simulink model "Brushless"  (R2020a)
settings: Solver=ode23  StartTime=0.0  StopTime=10.0  MaxStep=1e-2  RelTol=1e-3
undefined symbols (not defined in the file): CQ, I, Ke, Om, R, Ra, tau, V0, w_cm, zeta
libraries: fmu_me_lib x1, simulink x1
settings Model: Creator=Bob  LastModifiedBy=meagh
settings SFSimCC: CustomCodeUndefinedFunction=UseInterfaceOnly

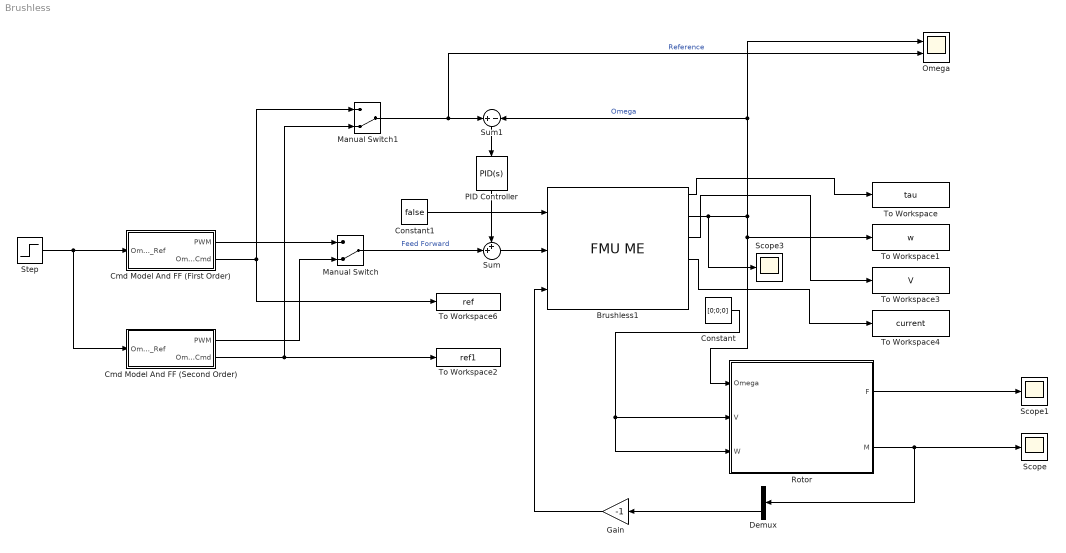
== system Brushless ==
  Brushless1 : fmu_me_lib/FMU ME  Description=Simulates an FMU for Model Exchange 1.0 or Model Exchange 2.0.  dummy=0
  Cmd Model And FF (First Order) : Subsystem
  Cmd Model And FF (Second Order) : Subsystem
  Constant : Constant  Value=[0;0;0]
  Constant1 : Constant  Value=false  OutDataTypeStr=boolean
  Demux : Demux  Outputs=3
  Gain : Gain  Gain=-1
  Manual Switch : ManualSwitch  CurrentSetting=0
  Manual Switch1 : ManualSwitch  CurrentSetting=0
  Omega : Scope  NumInputPorts=2
  PID Controller : simulink/Continuous/PID Controller  Controller=PID  Form=Parallel  TimeDomain=Continuous-time  UseExternalTs=off  SampleTime=-1  IntegratorMethod=Forward Euler  FilterMethod=Forward Euler  ControllerParametersSource=internal  P=0.0184*0.2  I=0.0184  D=0  UseFilter=on  N=100  TunerSelectOption=Transfer Function Based (PID Tuner App)  InitialConditionSource=internal  InitialConditionForIntegrator=0  InitialConditionForFilter=0  DifferentiatorICPrevScaledInput=0  ExternalReset=none  TrackingMode=off  Kt=1  LimitOutput=off  UpperSaturationLimit=inf  LowerSaturationLimit=-inf  LinearizeAsGain=on  AntiWindupMode=none  Kb=1  POutMin=[]  POutMax=[]  IOutMin=[]  IOutMax=[]  DOutMin=[]  DOutMax=[]  NOutMin=[]  NOutMax=[]  SumOutMin=[]  SumOutMax=[]  SaturationOutMin=[]  SaturationOutMax=[]  PParamMin=[]  PParamMax=[]  IParamMin=[]  IParamMax=[]  DParamMin=[]  DParamMax=[]  NParamMin=[]  NParamMax=[]  KbParamMin=[]  KbParamMax=[]  KtParamMin=[]  KtParamMax=[]  KbOutMin=[]  KbOutMax=[]  KtOutMin=[]  KtOutMax=[]  IntegratorOutMin=[]  IntegratorOutMax=[]  FilterOutMin=[]  FilterOutMax=[]  SumI1OutMin=[]  SumI1OutMax=[]  SumI2OutMin=[]  SumI2OutMax=[]  SumI3OutMin=[]  SumI3OutMax=[]  SumI4OutMin=[]  SumI4OutMax=[]  SumDOutMin=[]  SumDOutMax=[]  DifferentiatorOutMin=[]  DifferentiatorOutMax=[]  FilterDiffOutCoefMin=[]  FilterDiffOutCoefMax=[]  ReciprocalOutMin=[]  ReciprocalOutMax=[]  SumDenOutMin=[]  SumDenOutMax=[]  SumNumOutMin=[]  SumNumOutMax=[]  DivideOutMin=[]  DivideOutMax=[]  UdiffTsProdOutMin=[]  UdiffTsProdOutMax=[]  NTsProdOutMin=[]  NTsProdOutMax=[]  UintegralTsProdOutMin=[]  UintegralTsProdOutMax=[]  UngainTsProdOutMin=[]  UngainTsProdOutMax=[]  IntegratorContinuousStateAttributes=''  IntegratorStateMustResolveToSignalObject=off  IntegratorRTWStateStorageClass=Auto  FilterContinuousStateAttributes=''  FilterStateMustResolveToSignalObject=off  FilterRTWStateStorageClass=Auto  ParallelPVariant=InternalParameters  IdealPVariant=Disabled  IVariant=InternalParameters  DVariant=InternalParameters  IntegratorVariant=Continuous  SatVariant=Disabled  AWVariant=Passthrough  PCopyVariant=Disabled  TRVariant=Disabled  FdbkBlocksVariant=Forward  IdealPFdbkVariant=Disabled  SatFdbkVariant=Disabled  DerivativeFilterVariant=ContFilter  NVariant=InternalParameters  NCopyVariant=Disabled  FilterICVariant=InternalICsFilter  IntegratorICVariant=InternalICs  ExternalResetVariant=Disabled  TRSumVariant=Passthrough  SumFdbkVariant=Disabled  SumVariant=Sum_PID  TsampFilterVariant=InternalTs  TsampNgainVariant=Passthrough  TsampIntegralVariant=Passthrough
  Rotor : Subsystem
  Scope : Scope
  Scope1 : Scope
  Scope3 : Scope
  Step : Step  Time=5  Before=150  After=170  SampleTime=0
  Sum : Sum  Inputs=++|
  Sum1 : Sum  Inputs=+|-
  To Workspace : ToWorkspace  VariableName=tau  SaveFormat=Timeseries  SampleTime=-1
  To Workspace1 : ToWorkspace  VariableName=w  SaveFormat=Timeseries  SampleTime=-1
  To Workspace2 : ToWorkspace  VariableName=ref1  SaveFormat=Timeseries  SampleTime=-1
  To Workspace3 : ToWorkspace  VariableName=V  SaveFormat=Timeseries  SampleTime=-1
  To Workspace4 : ToWorkspace  VariableName=current  SaveFormat=Timeseries  SampleTime=-1
  To Workspace6 : ToWorkspace  VariableName=ref  SaveFormat=Timeseries  SampleTime=-1
  wires:
  Constant/1 -> Rotor/3(W), Rotor/2(V)
  Rotor/2(M) -> Demux/1, Scope/1
  Rotor/1(F) -> Scope1/1
  Demux/3 -> Gain/1
  Brushless1/2 -> Scope3/1, To Workspace1/1, Rotor/1(Omega), Omega/1, Sum1/2  "Omega"
  Step/1 -> Cmd Model And FF (Second Order)/1(Omega_Ref), Cmd Model And FF (First Order)/1(Omega_Ref)
  Cmd Model And FF (First Order)/1(PWM) -> Manual Switch/1
  Cmd Model And FF (Second Order)/1(PWM) -> Manual Switch/2
  Sum/1 -> Brushless1/2
  Manual Switch/1 -> Sum/2  "Feed Forward"
  Manual Switch1/1 -> Omega/2, Sum1/1  "Reference"
  Sum1/1 -> PID Controller/1
  PID Controller/1 -> Sum/1
  Cmd Model And FF (First Order)/2(Omega_Cmd) -> To Workspace6/1, Manual Switch1/1
  Cmd Model And FF (Second Order)/2(Omega_Cmd) -> To Workspace2/1, Manual Switch1/2
  Constant1/1 -> Brushless1/1
  Brushless1/1 -> To Workspace/1
  Brushless1/3 -> To Workspace3/1
  Brushless1/4 -> To Workspace4/1
  Gain/1 -> Brushless1/3

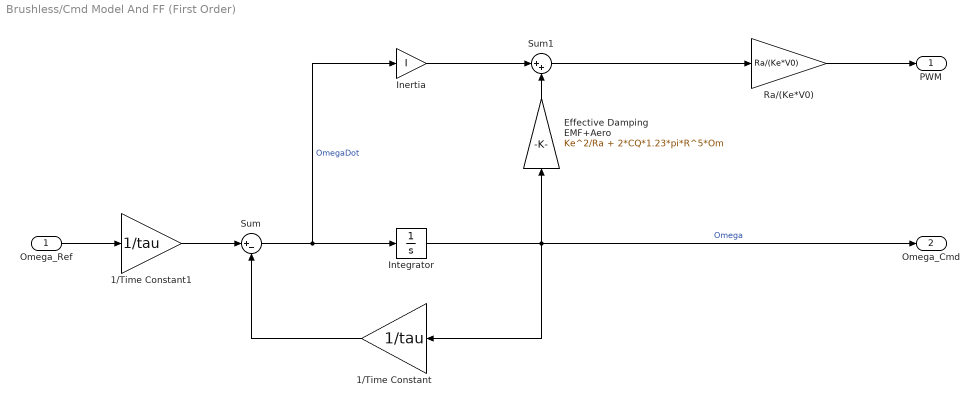
== system Brushless/Cmd Model And FF (First Order) ==
  Omega_Ref : Inport
  1/Time Constant : Gain  Gain=1/tau
  1/Time Constant1 : Gain  Gain=1/tau
  Effective Damping EMF+Aero : Gain  Gain=Ke^2/Ra + 2*CQ*1.23*pi*R^5*Om
  Inertia : Gain  Gain=I
  Integrator : Integrator
  Ra/(Ke*V0) : Gain  Gain=Ra/(Ke*V0)
  Sum : Sum  Inputs=|+-
  Sum1 : Sum  Inputs=|++
  PWM : Outport  VectorParamsAs1DForOutWhenUnconnected=off
  Omega_Cmd : Outport  Port=2  VectorParamsAs1DForOutWhenUnconnected=off
  wires:
  Omega_Ref/1 -> 1/Time Constant1/1
  1/Time Constant1/1 -> Sum/1
  Sum/1 -> Inertia/1, Integrator/1  "OmegaDot"
  1/Time Constant/1 -> Sum/2
  Integrator/1 -> Omega_Cmd/1, Effective Damping EMF+Aero/1, 1/Time Constant/1  "Omega"
  Ra/(Ke*V0)/1 -> PWM/1
  Sum1/1 -> Ra/(Ke*V0)/1
  Effective Damping EMF+Aero/1 -> Sum1/2
  Inertia/1 -> Sum1/1

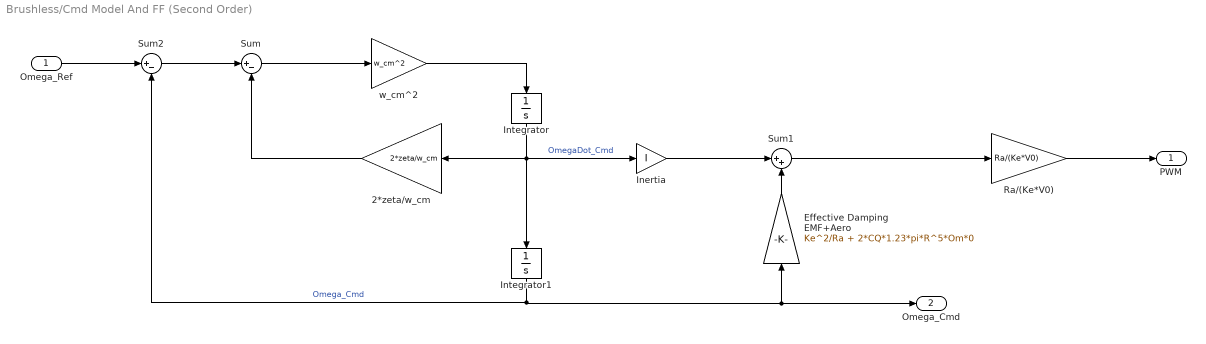
== system Brushless/Cmd Model And FF (Second Order) ==
  Omega_Ref : Inport
  2*zeta/w_cm : Gain  Gain=2*zeta/w_cm
  Effective Damping EMF+Aero : Gain  Gain=Ke^2/Ra + 2*CQ*1.23*pi*R^5*Om*0
  Inertia : Gain  Gain=I
  Integrator : Integrator
  Integrator1 : Integrator
  Ra/(Ke*V0) : Gain  Gain=Ra/(Ke*V0)
  Sum : Sum  Inputs=|+-
  Sum1 : Sum  Inputs=|++
  Sum2 : Sum  Inputs=|+-
  w_cm^2 : Gain  Gain=w_cm^2
  PWM : Outport  VectorParamsAs1DForOutWhenUnconnected=off
  Omega_Cmd : Outport  Port=2  VectorParamsAs1DForOutWhenUnconnected=off
  wires:
  Omega_Ref/1 -> Sum2/1
  Sum2/1 -> Sum/1
  2*zeta/w_cm/1 -> Sum/2
  Ra/(Ke*V0)/1 -> PWM/1
  Sum1/1 -> Ra/(Ke*V0)/1
  Effective Damping EMF+Aero/1 -> Sum1/2
  Inertia/1 -> Sum1/1
  Sum/1 -> w_cm^2/1
  w_cm^2/1 -> Integrator/1
  Integrator/1 -> Inertia/1, 2*zeta/w_cm/1, Integrator1/1  "OmegaDot_Cmd"
  Integrator1/1 -> Effective Damping EMF+Aero/1, Omega_Cmd/1, Sum2/2  "Omega_Cmd"

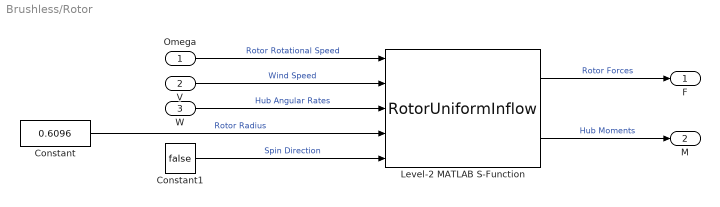
== system Brushless/Rotor ==
  Omega : Inport  OutDataTypeStr=double
  V : Inport  Port=2  OutDataTypeStr=double
  W : Inport  Port=3  OutDataTypeStr=double
  Constant : Constant  Value=0.6096
  Constant1 : Constant  Value=false  OutDataTypeStr=boolean
  Level-2 MATLAB S-Function : M-S-Function  FunctionName=RotorUniformInflow
  F : Outport  OutDataTypeStr=double  VectorParamsAs1DForOutWhenUnconnected=off
  M : Outport  Port=2  OutDataTypeStr=double  VectorParamsAs1DForOutWhenUnconnected=off
  wires:
  Level-2 MATLAB S-Function/2 -> M/1  "Hub Moments"
  Constant/1 -> Level-2 MATLAB S-Function/4  "Rotor Radius"
  Constant1/1 -> Level-2 MATLAB S-Function/5  "Spin Direction"
  Omega/1 -> Level-2 MATLAB S-Function/1  "Rotor Rotational Speed"
  V/1 -> Level-2 MATLAB S-Function/2  "Wind Speed"
  Level-2 MATLAB S-Function/1 -> F/1  "Rotor Forces"
  W/1 -> Level-2 MATLAB S-Function/3  "Hub Angular Rates"
